simulink model "Trimmodel"  (R2023b)
settings: Solver=ode4  StartTime=0.0  StopTime=100  FixedStep=1e-3  RelTol=1e-3
undefined symbols (not defined in the file or in its folder): Aeroparams, Aircraftparams, Atmosphereparams, Inertiaconstants, Initialconds, Propparams
libraries: simulink_extras x25
(part 2 of 3)

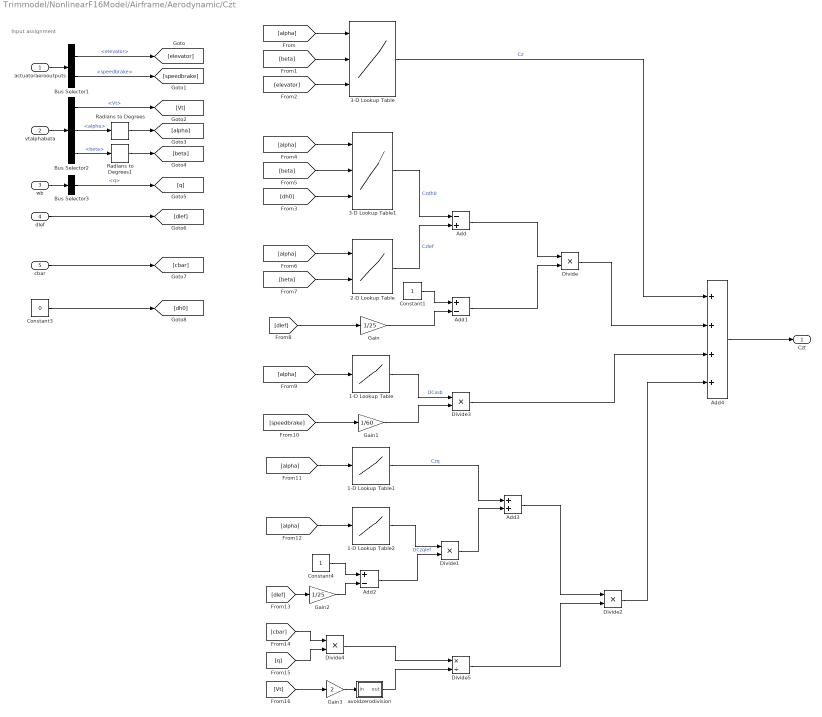
== system Trimmodel/NonlinearF16Model/Airframe/Aerodynamic/Czt ==
  note: Input assignment
  actuatoraerooutputs : Inport
  vtalphabeta : Inport  Port=2
  wb : Inport  Port=3
  dlef : Inport  Port=4
  cbar : Inport  Port=5
  1-D Lookup Table : Lookup_n-D  NumberOfTableDimensions=1  BreakpointsForDimension1=Aeroparams.alpha  Table=Aeroparams.DCzsb  InternalRulePriority=Speed  RndMeth=Simplest
  1-D Lookup Table1 : Lookup_n-D  NumberOfTableDimensions=1  BreakpointsForDimension1=Aeroparams.alpha  Table=Aeroparams.Czq  InternalRulePriority=Speed  RndMeth=Simplest
  1-D Lookup Table2 : Lookup_n-D  NumberOfTableDimensions=1  BreakpointsForDimension1=Aeroparams.alpha(1:14)  Table=Aeroparams.DCzqlef  InternalRulePriority=Speed  RndMeth=Simplest
  2-D Lookup Table : Lookup_n-D  BreakpointsForDimension1=Aeroparams.alpha(1:14)  BreakpointsForDimension2=Aeroparams.beta  Table=Aeroparams.Czlef  InternalRulePriority=Speed  RndMeth=Simplest
      settings: InputPortMap=u0,u1
  3-D Lookup Table : Lookup_n-D  NumberOfTableDimensions=3  BreakpointsForDimension1=Aeroparams.alpha  BreakpointsForDimension2=Aeroparams.beta  BreakpointsForDimension3=Aeroparams.dh  Table=Aeroparams.Cz  InternalRulePriority=Speed  RndMeth=Simplest
      settings: InputPortMap=u0,u1,u2
  3-D Lookup Table1 : Lookup_n-D  NumberOfTableDimensions=3  BreakpointsForDimension1=Aeroparams.alpha  BreakpointsForDimension2=Aeroparams.beta  BreakpointsForDimension3=Aeroparams.dh  Table=Aeroparams.Cz  InternalRulePriority=Speed  RndMeth=Simplest
      settings: InputPortMap=u0,u1,u2
  Add : Sum  Inputs=-+
  Add1 : Sum  Inputs=+-
  Add2 : Sum  Inputs=+-
  Add3 : Sum
  Add4 : Sum  Inputs=++++
  Bus Selector1 : BusSelector  OutputSignals=elevator,speedbrake
  Bus Selector2 : BusSelector  OutputSignals=Vt,alpha,beta
  Bus Selector3 : BusSelector  OutputSignals=q
  Constant1 : Constant
  Constant3 : Constant  Value=0
  Constant4 : Constant
  Divide{,1..4} (5 alike) : Product  Inputs=**
  Divide5 : Product  Inputs=*/
  Gain : Gain  Gain=1/25
  Gain1 : Gain  Gain=1/60
  Gain2 : Gain  Gain=1/25
  Gain3 : Gain  Gain=2
  Radians to Degrees : simulink_extras/Transformations/Radians to Degrees
  Radians to Degrees1 : simulink_extras/Transformations/Radians to Degrees
  avoidzerodivision : Subsystem
  Czt : Outport
  wires:
  Add4/1 -> Czt/1
  Divide2/1 -> Add4/4
  Divide3/1 -> Add4/3
  Divide5/1 -> Divide2/2
  Gain3/1 -> avoidzerodivision/1(in)
  Divide4/1 -> Divide5/1
  [Vt] -> Gain3/1
  [q] -> Divide4/2
  [cbar] -> Divide4/1
  Add3/1 -> Divide2/1
  Divide1/1 -> Add3/2
  1-D Lookup Table1/1 -> Add3/1  "Czq"
  Add2/1 -> Divide1/2
  1-D Lookup Table2/1 -> Divide1/1  "DCzqlef"
  Constant4/1 -> Add2/1
  Gain2/1 -> Add2/2
  [dlef] -> Gain2/1
  [alpha] -> 1-D Lookup Table2/1
  [alpha] -> 1-D Lookup Table1/1
  Gain1/1 -> Divide3/2
  1-D Lookup Table/1 -> Divide3/1  "DCxsb"
  [speedbrake] -> Gain1/1
  [alpha] -> 1-D Lookup Table/1
  [dlef] -> Gain/1
  [beta] -> 2-D Lookup Table/2
  [alpha] -> 2-D Lookup Table/1
  [alpha] -> 3-D Lookup Table1/1
  [beta] -> 3-D Lookup Table1/2
  Constant3/1 -> [dh0]
  [elevator] -> 3-D Lookup Table/3
  [beta] -> 3-D Lookup Table/2
  [alpha] -> 3-D Lookup Table/1
  dlef/1 -> [dlef]
  Bus Selector3/1 -> [q]  "<q>"
  Bus Selector2/3 -> Radians to Degrees1/1  "<beta>"
  Bus Selector2/2 -> Radians to Degrees/1  "<alpha>"
  Bus Selector2/1 -> [Vt]  "<Vt>"
  Bus Selector1/2 -> [speedbrake]  "<speedbrake>"
  Bus Selector1/1 -> [elevator]  "<elevator>"
  Divide/1 -> Add4/2
  Add1/1 -> Divide/2
  Add/1 -> Divide/1
  Gain/1 -> Add1/2
  Constant1/1 -> Add1/1
  3-D Lookup Table1/1 -> Add/1  "Czdh0"
  [dh0] -> 3-D Lookup Table1/3
  2-D Lookup Table/1 -> Add/2  "Czlef"
  3-D Lookup Table/1 -> Add4/1  "Cz"
  wb/1 -> Bus Selector3/1
  vtalphabeta/1 -> Bus Selector2/1
  actuatoraerooutputs/1 -> Bus Selector1/1
  cbar/1 -> [cbar]
  avoidzerodivision/1(out) -> Divide5/2
  Radians to Degrees/1 -> [alpha]
  Radians to Degrees1/1 -> [beta]

== system Trimmodel/NonlinearF16Model/Airframe/Aerodynamic/aeromodelcombineforcesandmoments ==
  Xa : Inport
  Za : Inport  Port=2
  Ma : Inport  Port=3
  Ya : Inport  Port=4
  Na : Inport  Port=5
  La : Inport  Port=6
  Outport : Outport
  Outport1 : Outport  Port=2
  Outport2 : Outport  Port=3
  Outport3 : Outport  Port=4
  Outport4 : Outport  Port=5
  Outport5 : Outport  Port=6
  wires:
  Ya/1 -> Outport1/1  "Ya"
  Xa/1 -> Outport/1  "Xa"
  Za/1 -> Outport2/1  "Za"
  La/1 -> Outport3/1  "La"
  Ma/1 -> Outport4/1  "Ma"
  Na/1 -> Outport5/1  "Na"

== system Trimmodel/NonlinearF16Model/Airframe/Aerodynamic/dlef ==
  vtalphabeta : Inport
  pressure : Inport  Port=2
  Add : Sum  Inputs=+-+
  Bus Selector : BusSelector  OutputSignals=alpha
  Bus Selector1 : BusSelector  OutputSignals=qbar,Ps
  Constant : Constant  Value=1.45
  Divide : Product  Inputs=*/
  Flapactuator : TransferFcn  Denominator=[0.136 1]
  Gain : Gain  Gain=1.38
  Gain1 : Gain  Gain=9.05
  Radians to Degrees : simulink_extras/Transformations/Radians to Degrees
  Rate Limiter : RateLimiter  RisingSlewLimit=25  FallingSlewLimit=-25
  Saturation : Saturate  UpperLimit=25  LowerLimit=0
  Transfer Fcn : TransferFcn  Numerator=[2 7.25]  Denominator=[1 7.25]
  avoidzerodivision : Subsystem
  dlef : Outport
  wires:
  vtalphabeta/1 -> Bus Selector/1
  pressure/1 -> Bus Selector1/1
  Bus Selector1/1 -> Divide/1  "<qbar>"
  Bus Selector1/2 -> avoidzerodivision/1(in)  "<Ps>"
  Bus Selector/1 -> Radians to Degrees/1  "<alpha>"
  Gain/1 -> Transfer Fcn/1
  Divide/1 -> Gain1/1
  Gain1/1 -> Add/2
  Transfer Fcn/1 -> Add/1
  Constant/1 -> Add/3
  Add/1 -> Saturation/1
  Saturation/1 -> Rate Limiter/1
  Rate Limiter/1 -> Flapactuator/1
  avoidzerodivision/1(out) -> Divide/2
  Radians to Degrees/1 -> Gain/1
  Flapactuator/1 -> dlef/1

== system Trimmodel/NonlinearF16Model/Airframe/Aerodynamic/qbarS ==
  pressure : Inport
  S : Inport  Port=2
  Bus Selector1 : BusSelector  OutputSignals=qbar
  Divide : Product  Inputs=**
  qbarS : Outport
  wires:
  pressure/1 -> Bus Selector1/1
  S/1 -> Divide/2  "S"
  Bus Selector1/1 -> Divide/1  "<qbar>"
  Divide/1 -> qbarS/1

== system Trimmodel/NonlinearF16Model/Airframe/Mass/massmodelgb ==
  note: Input assignment
  <phi> : Inport
  <theta> : Inport  Port=2
  <psi> : Inport  Port=3
  Bus Selector2 : BusSelector  OutputSignals=g0
  Constant1 : Constant  Value=Atmosphereparams  OutDataTypeStr=Bus: atmosphereparams
  Constant2 : Constant  Value=0
  Constant3 : Constant  Value=0
  Cos : Trigonometry  Operator=cos
  Cos1 : Trigonometry  Operator=cos
  Cos2 : Trigonometry
  Cos3 : Trigonometry
  Cos4 : Trigonometry  Operator=cos
  Cos5 : Trigonometry
  Firstrow : Subsystem
  Matrix Concatenate : Concatenate  NumInputs=3  Mode=Multidimensional array
  Matrix Multiply : Product  Multiplication=Matrix(*)
  Secondrow : Subsystem
  Thirdrow : Subsystem
  Vector Concatenate : Concatenate  NumInputs=3  Mode=Multidimensional array
  gb : Outport
  wires:
  <theta>/1 -> Cos3/1, Cos/1
  <psi>/1 -> Cos1/1, Cos2/1
  <phi>/1 -> Cos5/1, Cos4/1
  Cos4/1 -> [cosphi]
  Cos5/1 -> [sinphi]
  Cos/1 -> [costheta]
  Cos3/1 -> [sintheta]
  Cos1/1 -> [cospsi]
  Cos2/1 -> [sinpsi]
  Firstrow/1(firstrow) -> Matrix Concatenate/1
  Secondrow/1(secondrow) -> Matrix Concatenate/2
  Thirdrow/1(thirdrow) -> Matrix Concatenate/3
  [sinpsi] -> Secondrow/6(sinpsi)
  [cosphi] -> Thirdrow/1(cosphi)
  [cospsi] -> Secondrow/5(cospsi)
  [sinphi] -> Thirdrow/2(sinphi)
  [cospsi] -> Thirdrow/5(cospsi)
  [sinpsi] -> Firstrow/4(sinpsi)
  [costheta] -> Thirdrow/3(costheta)
  [sinpsi] -> Thirdrow/6(sinpsi)
  [cosphi] -> Secondrow/1(cosphi)
  [sintheta] -> Thirdrow/4(sintheta)
  [sinphi] -> Secondrow/2(sinphi)
  [costheta] -> Firstrow/1(costheta)
  [costheta] -> Secondrow/3(costheta)
  [cospsi] -> Firstrow/3(cospsi)
  [sintheta] -> Secondrow/4(sintheta)
  [sintheta] -> Firstrow/2(sintheta)
  Constant1/1 -> Bus Selector2/1
  Bus Selector2/1 -> [g0]  "<g0>"
  Matrix Concatenate/1 -> Matrix Multiply/1
  Constant3/1 -> Vector Concatenate/2
  Constant2/1 -> Vector Concatenate/1
  [g0] -> Vector Concatenate/3
  Vector Concatenate/1 -> Matrix Multiply/2
  Matrix Multiply/1 -> gb/1  "gxgygz"

== system Trimmodel/NonlinearF16Model/Airframe/Propulsion/Padot ==
  Pc : Inport
  Add : Sum  Inputs=+-
  Bus Selector : BusSelector  OutputSignals=Paic
  Constant : Constant  Value=Initialconds  OutDataTypeStr=Bus: initialconds
  Divide : Product  Inputs=**
  PA : Integrator  InitialConditionSource=external
  propmodeltauPc : Subsystem
  Pa : Outport
  wires:
  PA/1 -> propmodeltauPc/2(Pa), Pa/1, Add/2  "Pa"
  Constant/1 -> Bus Selector/1
  Bus Selector/1 -> PA/2  "<Paic>"
  Pc/1 -> propmodeltauPc/1(Pc)
  propmodeltauPc/2(Outport) -> Add/1
  propmodeltauPc/1(Outport1) -> Divide/1
  Add/1 -> Divide/2
  Divide/1 -> PA/1  "Padot"

== system Trimmodel/NonlinearF16Model/Airframe/Propulsion/Tgear ==
  thrust : Inport
  Add : Sum  Inputs=+-
  Constant : Constant  Value=217.38
  Constant1 : Constant  Value=64.94
  Constant2 : Constant  Value=117.38
  Divide : Product  Inputs=**
  Divide1 : Product  Inputs=**
  Saturation : Saturate  UpperLimit=100  LowerLimit=0
  Switch : Switch  Criteria=u2 > Threshold  Threshold=0.77  SaturateOnIntegerOverflow=off  InputSameDT=off
  Pc : Outport
  wires:
  thrust/1 -> Switch/2, Divide1/1, Divide/2
  Constant/1 -> Divide/1
  Divide1/1 -> Switch/3
  Constant1/1 -> Divide1/2
  Switch/1 -> Saturation/1
  Saturation/1 -> Pc/1
  Divide/1 -> Add/1
  Constant2/1 -> Add/2
  Add/1 -> Switch/1

== system Trimmodel/NonlinearF16Model/Airframe/Propulsion/propmodelTidleTmil ==
  note: Input assignment
  Pa : Inport
  M : Inport  Port=2
  h : Inport  Port=3
  Add : Sum  Inputs=-+
  Add1 : Sum
  Divide : Product  Inputs=**
  Gain : Gain  Gain=1/50
  Tidle : Lookup_n-D  BreakpointsForDimension1=Propparams.M  BreakpointsForDimension2=Propparams.h  Table=Propparams.Tidle  InternalRulePriority=Speed  RndMeth=Simplest
      settings: InputPortMap=u0,u1
  Tmil : Lookup_n-D  BreakpointsForDimension1=Propparams.M  BreakpointsForDimension2=Propparams.h  Table=Propparams.Tmil  InternalRulePriority=Speed  RndMeth=Simplest
      settings: InputPortMap=u0,u1
  Tx : Outport
  wires:
  Tmil/1 -> Add/2
  Tidle/1 -> Add1/1, Add/1
  M/1 -> [M]
  Pa/1 -> [Pa]
  h/1 -> [h]
  [M] -> Tidle/1
  [h] -> Tidle/2
  [M] -> Tmil/1
  [h] -> Tmil/2
  Add/1 -> Divide/1
  [Pa] -> Gain/1
  Gain/1 -> Divide/2
  Divide/1 -> Add1/2
  Add1/1 -> Tx/1

== system Trimmodel/NonlinearF16Model/Airframe/Propulsion/propmodelTmilTmax ==
  note: Input assignment
  M : Inport
  h : Inport  Port=2
  Pa : Inport  Port=3
  Add : Sum  Inputs=-+
  Add1 : Sum
  Add2 : Sum  Inputs=-+
  Constant : Constant  Value=50
  Divide : Product  Inputs=**
  Gain1 : Gain  Gain=1/50
  Tmax : Lookup_n-D  BreakpointsForDimension1=Propparams.M  BreakpointsForDimension2=Propparams.h  Table=Propparams.Tmax  InternalRulePriority=Speed  RndMeth=Simplest
      settings: InputPortMap=u0,u1
  Tmil : Lookup_n-D  BreakpointsForDimension1=Propparams.M  BreakpointsForDimension2=Propparams.h  Table=Propparams.Tmil  InternalRulePriority=Speed  RndMeth=Simplest
      settings: InputPortMap=u0,u1
  Tx : Outport
  wires:
  Add1/1 -> Tx/1
  Divide/1 -> Add1/2
  Gain1/1 -> Divide/2
  [Pa] -> Add2/2
  Add/1 -> Divide/1
  [h] -> Tmax/2
  [M] -> Tmax/1
  [h] -> Tmil/2
  [M] -> Tmil/1
  h/1 -> [h]
  Pa/1 -> [Pa]
  M/1 -> [M]
  Tmil/1 -> Add/1, Add1/1
  Tmax/1 -> Add/2
  Constant/1 -> Add2/1
  Add2/1 -> Gain1/1

== system Trimmodel/NonlinearF16Model/Simframe/Environmentmodel/Vtalphabeta ==
  note: Input assignment
  disturbances : Inport
  bodyvelocities : Inport  Port=2
  Add : Sum  Inputs=-+
  Add1 : Sum  Inputs=-+
  Add2 : Sum  Inputs=-+
  Add3 : Sum  Inputs=+++
  Asin : Trigonometry  Operator=asin
  Atan2 : Trigonometry  Operator=atan2
  Bus Selector : BusSelector  OutputSignals=windz,windy,windx
  Bus Selector1 : BusSelector  OutputSignals=u,v,w
  Divide : Product  Inputs=*/
  Square : Math  Operator=square
  Square Root : Sqrt
  Square1 : Math  Operator=square
  Square2 : Math  Operator=square
  avoidzerodivision : Subsystem
  Vt : Outport
  alpha : Outport  Port=2
  beta : Outport  Port=3
  wires:
  avoidzerodivision/1(out) -> Divide/2
  Asin/1 -> beta/1  "beta"
  Divide/1 -> Asin/1
  [vt] -> Divide/1
  Atan2/1 -> alpha/1  "alpha"
  [ut] -> Atan2/2
  [wt] -> Atan2/1
  Square Root/1 -> avoidzerodivision/1(in), Vt/1  "Vt"
  Add3/1 -> Square Root/1
  Square2/1 -> Add3/3
  Square/1 -> Add3/1
  Square1/1 -> Add3/2
  [wt] -> Square2/1
  [vt] -> Square1/1
  [ut] -> Square/1
  Add2/1 -> [wt]
  Add1/1 -> [vt]
  Add/1 -> [ut]
  Bus Selector/3 -> Add/1  "<windx>"
  Bus Selector/2 -> Add1/1  "<windy>"
  Bus Selector/1 -> Add2/1  "<windz>"
  Bus Selector1/3 -> Add2/2  "<w>"
  Bus Selector1/2 -> Add1/2  "<v>"
  Bus Selector1/1 -> Add/2  "<u>"
  bodyvelocities/1 -> Bus Selector1/1
  disturbances/1 -> Bus Selector/1

== system Trimmodel/NonlinearF16Model/Simframe/Environmentmodel/envmodelTM ==
  note: Input assignment
  T0 : Inport
  L : Inport  Port=2
  h : Inport  Port=3
  gamma : Inport  Port=4
  R : Inport  Port=5
  Vt : Inport  Port=6
  Add : Sum  Inputs=+-
  Add1 : Sum  Inputs=+-
  Constant1 : Constant  Value=11000
  Divide : Product  Inputs=**
  Divide1 : Product  Inputs=**
  Divide15 : Product  Inputs=*/
  Divide2 : Product  Inputs=***
  Square Root : Sqrt
  Switch : Switch  Threshold=11000  SaturateOnIntegerOverflow=off  InputSameDT=off
  T : Outport
  M : Outport  Port=2
  wires:
  gamma/1 -> Divide2/2  "gamma"
  R/1 -> Divide2/3  "R"
  Square Root/1 -> Divide15/2  "a"
  Vt/1 -> Divide15/1
  Divide2/1 -> Square Root/1
  Divide15/1 -> M/1  "M"
  Switch/1 -> Divide2/1, T/1  "T"
  h/1 -> [h]
  L/1 -> [L]
  T0/1 -> [T0]
  [h] -> Switch/2
  Divide/1 -> Add/2
  Divide1/1 -> Add1/2
  Add/1 -> Switch/1  "T11"
  Constant1/1 -> Divide/2
  [T0] -> Add1/1
  [T0] -> Add/1
  [h] -> Divide1/2
  [L] -> Divide/1
  [L] -> Divide1/1
  Add1/1 -> Switch/3  "T"

== system Trimmodel/NonlinearF16Model/Simframe/Environmentmodel/envmodelqbarPs ==
  rho : Inport
  R : Inport  Port=2
  T : Inport  Port=3
  Vt : Inport  Port=4
  Constant3 : Constant  Value=1/2
  Divide13 : Product  Inputs=***
  Divide14 : Product  Inputs=***
  Square : Math  Operator=square
  qbar : Outport
  Ps : Outport  Port=2
  wires:
  Constant3/1 -> Divide14/1
  Square/1 -> Divide14/2
  T/1 -> Divide13/3
  rho/1 -> Divide14/3, Divide13/1
  R/1 -> Divide13/2
  Divide13/1 -> Ps/1  "Ps"
  Vt/1 -> Square/1
  Divide14/1 -> qbar/1  "qbar"

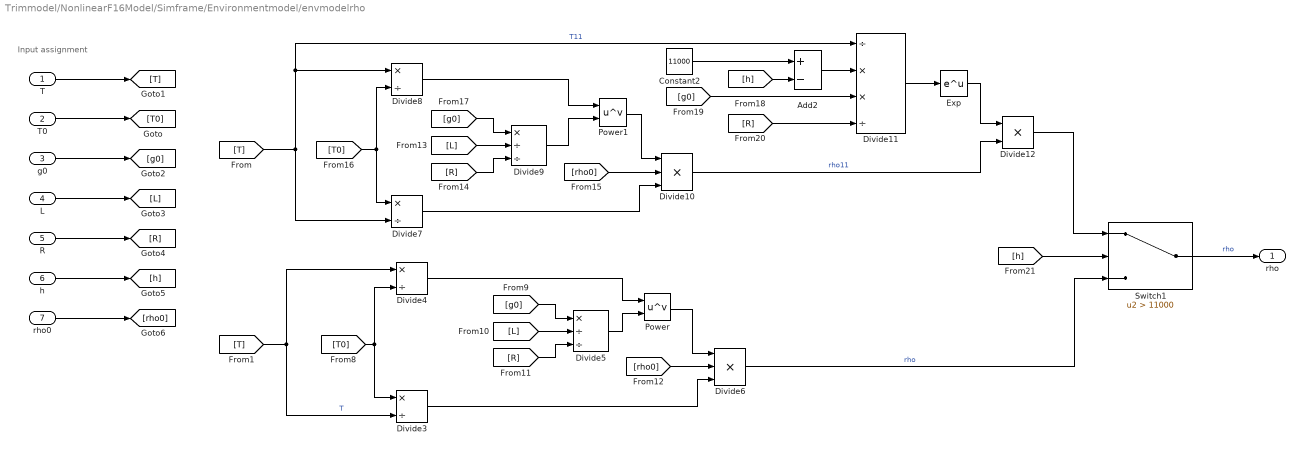
== system Trimmodel/NonlinearF16Model/Simframe/Environmentmodel/envmodelrho ==
  note: Input assignment
  T : Inport
  T0 : Inport  Port=2
  g0 : Inport  Port=3
  L : Inport  Port=4
  R : Inport  Port=5
  h : Inport  Port=6
  rho0 : Inport  Port=7
  Add2 : Sum  Inputs=+-
  Constant2 : Constant  Value=11000
  Divide10 : Product  Inputs=***
  Divide11 : Product  Inputs=/**/
  Divide12 : Product  Inputs=**
  Divide{3..4,7..8} (4 alike) : Product  Inputs=*/
  Divide5 : Product  Inputs=*//
  Divide6 : Product  Inputs=***
  Divide9 : Product  Inputs=*//
  Exp : Math
  Power : Math  Operator=pow
  Power1 : Math  Operator=pow
  Switch1 : Switch  Criteria=u2 > Threshold  Threshold=11000  SaturateOnIntegerOverflow=off  InputSameDT=off
  rho : Outport
  wires:
  Switch1/1 -> rho/1  "rho"
  [h] -> Switch1/2
  rho0/1 -> [rho0]
  h/1 -> [h]
  R/1 -> [R]
  L/1 -> [L]
  g0/1 -> [g0]
  T/1 -> [T]
  T0/1 -> [T0]
  Divide4/1 -> Power/1
  [T0] -> Divide3/1, Divide4/2
  [L] -> Divide5/2
  [g0] -> Divide5/1
  Divide3/1 -> Divide6/3
  [rho0] -> Divide6/2
  [T] -> Divide3/2, Divide4/1  "T"
  Divide6/1 -> Switch1/3  "rho"
  Divide5/1 -> Power/2
  [R] -> Divide5/3
  Power/1 -> Divide6/1
  Exp/1 -> Divide12/1
  Add2/1 -> Divide11/2
  Divide11/1 -> Exp/1
  [g0] -> Divide9/1
  [T] -> Divide7/2, Divide8/1, Divide11/1  "T11"
  [rho0] -> Divide10/2
  [L] -> Divide9/2
  Constant2/1 -> Add2/1
  Divide8/1 -> Power1/1
  Divide9/1 -> Power1/2
  [R] -> Divide11/4
  [R] -> Divide9/3
  Divide10/1 -> Divide12/2  "rho11"
  [T0] -> Divide7/1, Divide8/2
  Power1/1 -> Divide10/1
  [h] -> Add2/2
  [g0] -> Divide11/3
  Divide7/1 -> Divide10/3
  Divide12/1 -> Switch1/1

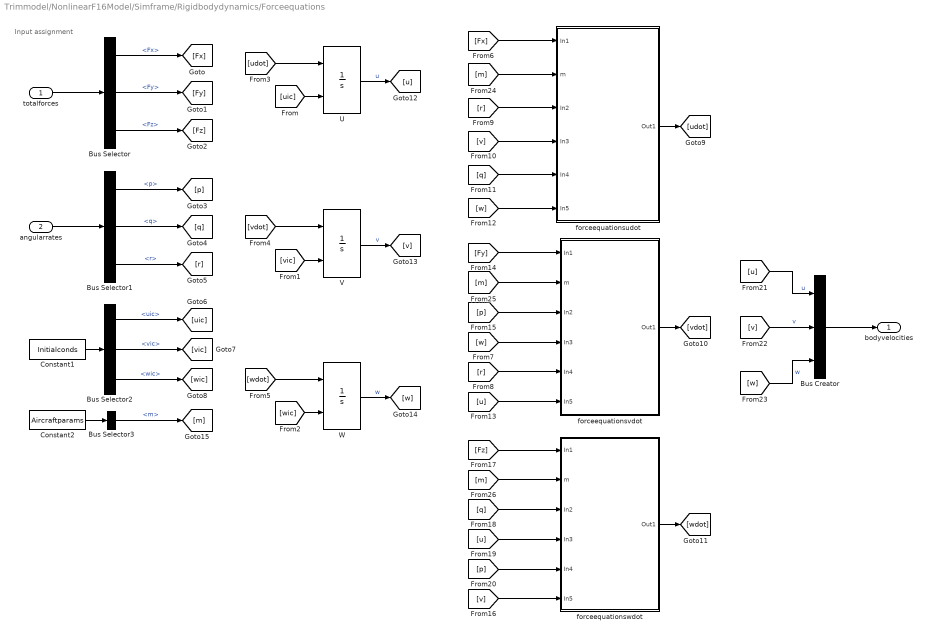
== system Trimmodel/NonlinearF16Model/Simframe/Rigidbodydynamics/Forceequations ==
  note: Input assignment
  totalforces : Inport
  angularrates : Inport  Port=2
  Bus Creator : BusCreator  Inputs=3  OutDataTypeStr=Bus: bodyvelocities
  Bus Selector : BusSelector  OutputSignals=Fx,Fy,Fz
  Bus Selector1 : BusSelector  OutputSignals=p,q,r
  Bus Selector2 : BusSelector  OutputSignals=uic,vic,wic
  Bus Selector3 : BusSelector  OutputSignals=m
  Constant1 : Constant  Value=Initialconds  OutDataTypeStr=Bus: initialconds
  Constant2 : Constant  Value=Aircraftparams  OutDataTypeStr=Bus: aircraftparams
  U : Integrator  InitialConditionSource=external
  V : Integrator  InitialConditionSource=external
  W : Integrator  InitialConditionSource=external
  forceequationsudot : Subsystem
  forceequationsvdot : Subsystem
  forceequationswdot : Subsystem
  bodyvelocities : Outport  OutDataTypeStr=Bus: bodyvelocities
  wires:
  totalforces/1 -> Bus Selector/1
  angularrates/1 -> Bus Selector1/1
  Bus Selector/1 -> [Fx]  "<Fx>"
  Bus Selector/2 -> [Fy]  "<Fy>"
  Bus Selector/3 -> [Fz]  "<Fz>"
  Bus Selector1/1 -> [p]  "<p>"
  Bus Selector1/2 -> [q]  "<q>"
  Bus Selector1/3 -> [r]  "<r>"
  Constant1/1 -> Bus Selector2/1
  Bus Selector2/1 -> [uic]  "<uic>"
  Bus Selector2/2 -> [vic]  "<vic>"
  Bus Selector2/3 -> [wic]  "<wic>"
  [uic] -> U/2
  [vic] -> V/2
  [wic] -> W/2
  forceequationsudot/1(Out1) -> [udot]
  [udot] -> U/1
  [vdot] -> V/1
  [wdot] -> W/1
  U/1 -> [u]  "u"
  V/1 -> [v]  "v"
  W/1 -> [w]  "w"
  [Fx] -> forceequationsudot/1(In1)
  [r] -> forceequationsudot/3(In2)
  [v] -> forceequationsudot/4(In3)
  [q] -> forceequationsudot/5(In4)
  [w] -> forceequationsudot/6(In5)
  [u] -> forceequationsvdot/6(In5)
  [r] -> forceequationsvdot/5(In4)
  [w] -> forceequationsvdot/4(In3)
  [p] -> forceequationsvdot/3(In2)
  [Fy] -> forceequationsvdot/1(In1)
  forceequationsvdot/1(Out1) -> [vdot]
  forceequationswdot/1(Out1) -> [wdot]
  [Fz] -> forceequationswdot/1(In1)
  [q] -> forceequationswdot/3(In2)
  [u] -> forceequationswdot/4(In3)
  [p] -> forceequationswdot/5(In4)
  [v] -> forceequationswdot/6(In5)
  [v] -> Bus Creator/2  "v"
  [u] -> Bus Creator/1  "u"
  [w] -> Bus Creator/3  "w"
  Bus Creator/1 -> bodyvelocities/1
  Constant2/1 -> Bus Selector3/1
  Bus Selector3/1 -> [m]  "<m>"
  [m] -> forceequationsudot/2(m)
  [m] -> forceequationsvdot/2(m)
  [m] -> forceequationswdot/2(m)

== system Trimmodel/NonlinearF16Model/Simframe/Rigidbodydynamics/Kinematicequations ==
  note: Input assignment
  angularrates : Inport
  Bus Creator : BusCreator  Inputs=3  OutDataTypeStr=Bus: eulerangles
  Bus Selector1 : BusSelector  OutputSignals=phiic,thetaic,psiic
  Constant : Constant  Value=Initialconds  OutDataTypeStr=Bus: initialconds
  Eulerlimitations : Subsystem
  PHI : Integrator  InitialConditionSource=external  WrapState=on
  PSI : Integrator  InitialConditionSource=external  WrapState=on
  THETA : Integrator  InitialConditionSource=external  WrapState=on
  kinematicequationseulerdot : Subsystem
  eulerangles : Outport  OutDataTypeStr=Bus: eulerangles
  wires:
  Eulerlimitations/3(Outport1) -> Bus Creator/3
  Eulerlimitations/1(<phi>) -> Bus Creator/1
  Eulerlimitations/2(Outport) -> Bus Creator/2
  [psi] -> Eulerlimitations/3(psi)
  [theta] -> Eulerlimitations/2(theta)
  [phi] -> Eulerlimitations/1(phi)
  PSI/1 -> [psi]  "psi"
  angularrates/1 -> kinematicequationseulerdot/2(angularrates)
  kinematicequationseulerdot/3(psidot) -> PSI/1
  kinematicequationseulerdot/2(thetadot) -> THETA/1
  kinematicequationseulerdot/1(phidot) -> PHI/1
  THETA/1 -> [theta], kinematicequationseulerdot/3(theta)  "theta"
  PHI/1 -> kinematicequationseulerdot/1(phi), [phi]  "phi"
  Bus Creator/1 -> eulerangles/1
  [psiic] -> PSI/2
  [thetaic] -> THETA/2
  [phiic] -> PHI/2
  Bus Selector1/3 -> [psiic]  "<psiic>"
  Bus Selector1/2 -> [thetaic]  "<thetaic>"
  Bus Selector1/1 -> [phiic]  "<phiic>"
  Constant/1 -> Bus Selector1/1

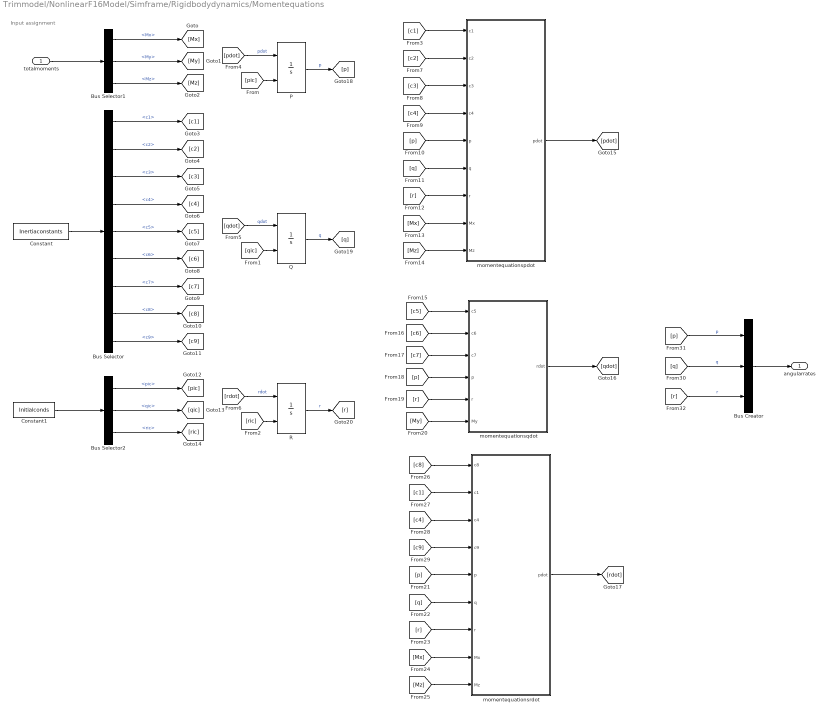
== system Trimmodel/NonlinearF16Model/Simframe/Rigidbodydynamics/Momentequations ==
  note: Input assignment
  totalmoments : Inport
  Bus Creator : BusCreator  Inputs=3  OutDataTypeStr=Bus: angularrates
  Bus Selector : BusSelector  OutputSignals=c1,c2,c3,c4,c5,c6,c7,c8,c9
  Bus Selector1 : BusSelector  OutputSignals=Mx,My,Mz
  Bus Selector2 : BusSelector  OutputSignals=pic,qic,ric
  Constant : Constant  Value=Inertiaconstants  OutDataTypeStr=Bus: inertiaconstants
  Constant1 : Constant  Value=Initialconds  OutDataTypeStr=Bus: initialconds
  P : Integrator  InitialConditionSource=external
  Q : Integrator  InitialConditionSource=external
  R : Integrator  InitialConditionSource=external
  momentequationspdot : Subsystem
  momentequationsqdot : Subsystem
  momentequationsrdot : Subsystem
  angularrates : Outport  OutDataTypeStr=Bus: angularrates
  wires:
  Constant/1 -> Bus Selector/1
  totalmoments/1 -> Bus Selector1/1
  Bus Selector1/1 -> [Mx]  "<Mx>"
  Bus Selector1/2 -> [My]  "<My>"
  Bus Selector1/3 -> [Mz]  "<Mz>"
  Bus Selector/1 -> [c1]  "<c1>"
  Bus Selector/2 -> [c2]  "<c2>"
  Bus Selector/3 -> [c3]  "<c3>"
  Bus Selector/4 -> [c4]  "<c4>"
  Bus Selector/5 -> [c5]  "<c5>"
  Bus Selector/6 -> [c6]  "<c6>"
  Bus Selector/7 -> [c7]  "<c7>"
  Bus Selector/8 -> [c8]  "<c8>"
  Bus Selector/9 -> [c9]  "<c9>"
  Constant1/1 -> Bus Selector2/1
  Bus Selector2/1 -> [pic]  "<pic>"
  Bus Selector2/2 -> [qic]  "<qic>"
  Bus Selector2/3 -> [ric]  "<ric>"
  [pdot] -> P/1  "pdot"
  [qdot] -> Q/1  "qdot"
  [rdot] -> R/1  "rdot"
  [pic] -> P/2
  [qic] -> Q/2
  [ric] -> R/2
  momentequationspdot/1(pdot) -> [pdot]
  momentequationsqdot/1(rdot) -> [qdot]
  P/1 -> [p]  "p"
  Q/1 -> [q]  "q"
  R/1 -> [r]  "r"
  [c1] -> momentequationspdot/1(c1)
  [c2] -> momentequationspdot/2(c2)
  [c3] -> momentequationspdot/3(c3)
  [c4] -> momentequationspdot/4(c4)
  [p] -> momentequationspdot/5(p)
  [q] -> momentequationspdot/6(q)
  [r] -> momentequationspdot/7(r)
  [Mx] -> momentequationspdot/8(Mx)
  [Mz] -> momentequationspdot/9(Mz)
  [c5] -> momentequationsqdot/1(c5)
  [c6] -> momentequationsqdot/2(c6)
  [c7] -> momentequationsqdot/3(c7)
  [p] -> momentequationsqdot/4(p)
  [r] -> momentequationsqdot/5(r)
  [My] -> momentequationsqdot/6(My)
  [Mz] -> momentequationsrdot/9(Mz)
  [Mx] -> momentequationsrdot/8(Mx)
  [r] -> momentequationsrdot/7(r)
  [q] -> momentequationsrdot/6(q)
  [p] -> momentequationsrdot/5(p)
  [c9] -> momentequationsrdot/4(c9)
  [c4] -> momentequationsrdot/3(c4)
  [c1] -> momentequationsrdot/2(c1)
  [c8] -> momentequationsrdot/1(c8)
  momentequationsrdot/1(pdot) -> [rdot]
  [q] -> Bus Creator/2  "q"
  [p] -> Bus Creator/1  "p"
  [r] -> Bus Creator/3  "r"
  Bus Creator/1 -> angularrates/1

== system Trimmodel/NonlinearF16Model/Simframe/Rigidbodydynamics/Navigationequations ==
  note: Input assignment
  bodyvelocities : Inport
  eulerangles : Inport  Port=2
  Bus Creator : BusCreator  Inputs=3  OutDataTypeStr=Bus: positions
  Bus Selector : BusSelector  OutputSignals=u,v,w
  Bus Selector1 : BusSelector  OutputSignals=phi,theta,psi
  Bus Selector2 : BusSelector  OutputSignals=xeic,yeic,zeic
  Constant : Constant  Value=Initialconds  OutDataTypeStr=Bus: initialconds
  Matrix Multiply : Product  Multiplication=Matrix(*)
  Selector : Selector  InputPortWidth=3  IndexOptions=Index vector (dialog)  Indices=1  OutputSizes=1
  Selector1 : Selector  InputPortWidth=3  IndexOptions=Index vector (dialog)  Indices=2  OutputSizes=1
  Selector2 : Selector  InputPortWidth=3  IndexOptions=Index vector (dialog)  Indices=3  OutputSizes=1
  Vector Concatenate : Concatenate  NumInputs=3  Mode=Multidimensional array
  XE : Integrator  InitialConditionSource=external
  YE : Integrator  InitialConditionSource=external
  ZE : Integrator  InitialConditionSource=external
  navigationequationstfmatrix : Subsystem
  positions : Outport  OutDataTypeStr=Bus: positions
  wires:
  bodyvelocities/1 -> Bus Selector/1
  Bus Selector1/2 -> navigationequationstfmatrix/2(<theta>)  "<theta>"
  Bus Selector1/1 -> navigationequationstfmatrix/1(<phi>)  "<phi>"
  Bus Selector1/3 -> navigationequationstfmatrix/3(<psi>)  "<psi>"
  Constant/1 -> Bus Selector2/1
  eulerangles/1 -> Bus Selector1/1
  Bus Selector/2 -> Vector Concatenate/2  "<v>"
  Bus Selector/3 -> Vector Concatenate/3  "<w>"
  Bus Selector/1 -> Vector Concatenate/1  "<u>"
  navigationequationstfmatrix/1(transformationmatrix) -> Matrix Multiply/1
  Vector Concatenate/1 -> Matrix Multiply/2
  Matrix Multiply/1 -> Selector2/1, Selector1/1, Selector/1
  Bus Selector2/1 -> [xeic]  "<xeic>"
  Bus Selector2/2 -> [yeic]  "<yeic>"
  Bus Selector2/3 -> [zeic]  "<zeic>"
  Selector/1 -> XE/1  "xedot"
  [xeic] -> XE/2
  Selector1/1 -> YE/1  "yedot"
  [yeic] -> YE/2
  Selector2/1 -> ZE/1  "zedot"
  [zeic] -> ZE/2
  YE/1 -> Bus Creator/2  "ye"
  XE/1 -> Bus Creator/1  "xe"
  ZE/1 -> Bus Creator/3  "ze"
  Bus Creator/1 -> positions/1

== system Trimmodel/NonlinearF16Model/Airframe/Aerodynamic/Clt/avoidzerodivision ==
  in : Inport
  Constant : Constant  Value=eps
  Switch : Switch  Criteria=u2 ~= 0  SaturateOnIntegerOverflow=off  InputSameDT=off
  out : Outport
  wires:
  in/1 -> Switch/1, Switch/2
  Constant/1 -> Switch/3
  Switch/1 -> out/1

== system Trimmodel/NonlinearF16Model/Airframe/Aerodynamic/Cmt/avoidzerodivision ==
  in : Inport
  Constant : Constant  Value=eps
  Switch : Switch  Criteria=u2 ~= 0  SaturateOnIntegerOverflow=off  InputSameDT=off
  out : Outport
  wires:
  in/1 -> Switch/1, Switch/2
  Constant/1 -> Switch/3
  Switch/1 -> out/1

== system Trimmodel/NonlinearF16Model/Airframe/Aerodynamic/Cnt/avoidzerodivision ==
  in : Inport
  Constant : Constant  Value=eps
  Switch : Switch  Criteria=u2 ~= 0  SaturateOnIntegerOverflow=off  InputSameDT=off
  out : Outport
  wires:
  in/1 -> Switch/1, Switch/2
  Constant/1 -> Switch/3
  Switch/1 -> out/1

== system Trimmodel/NonlinearF16Model/Airframe/Aerodynamic/Cxt/avoidzerodivision ==
  in : Inport
  Constant : Constant  Value=eps
  Switch : Switch  Criteria=u2 ~= 0  SaturateOnIntegerOverflow=off  InputSameDT=off
  out : Outport
  wires:
  in/1 -> Switch/1, Switch/2
  Constant/1 -> Switch/3
  Switch/1 -> out/1

== system Trimmodel/NonlinearF16Model/Airframe/Aerodynamic/Cyt/avoidzerodivision ==
  in : Inport
  Constant : Constant  Value=eps
  Switch : Switch  Criteria=u2 ~= 0  SaturateOnIntegerOverflow=off  InputSameDT=off
  out : Outport
  wires:
  in/1 -> Switch/1, Switch/2
  Constant/1 -> Switch/3
  Switch/1 -> out/1

== system Trimmodel/NonlinearF16Model/Airframe/Aerodynamic/Czt/avoidzerodivision ==
  in : Inport
  Constant : Constant  Value=eps
  Switch : Switch  Criteria=u2 ~= 0  SaturateOnIntegerOverflow=off  InputSameDT=off
  out : Outport
  wires:
  in/1 -> Switch/1, Switch/2
  Constant/1 -> Switch/3
  Switch/1 -> out/1

== system Trimmodel/NonlinearF16Model/Airframe/Aerodynamic/dlef/avoidzerodivision ==
  in : Inport
  Constant : Constant  Value=eps
  Switch : Switch  Criteria=u2 ~= 0  SaturateOnIntegerOverflow=off  InputSameDT=off
  out : Outport
  wires:
  in/1 -> Switch/1, Switch/2
  Constant/1 -> Switch/3
  Switch/1 -> out/1

== system Trimmodel/NonlinearF16Model/Airframe/Mass/massmodelgb/Firstrow ==
  note: Input assignment
  costheta : Inport
  sintheta : Inport  Port=2
  cospsi : Inport  Port=3
  sinpsi : Inport  Port=4
  Divide : Product  Inputs=**
  Divide2 : Product  Inputs=**
  Gain : Gain  Gain=-1
  Vector Concatenate : Concatenate  NumInputs=3  Mode=Multidimensional array  ConcatenateDimension=2
  firstrow : Outport
  wires:
  costheta/1 -> [costheta]
  sintheta/1 -> [sintheta]
  cospsi/1 -> [cospsi]
  sinpsi/1 -> [sinpsi]
  [costheta] -> Divide/1
  [cospsi] -> Divide/2
  [costheta] -> Divide2/1
  [sinpsi] -> Divide2/2
  [sintheta] -> Gain/1
  Divide/1 -> Vector Concatenate/1
  Divide2/1 -> Vector Concatenate/2
  Gain/1 -> Vector Concatenate/3
  Vector Concatenate/1 -> firstrow/1

== system Trimmodel/NonlinearF16Model/Airframe/Mass/massmodelgb/Secondrow ==
  note: Input assignment
  cosphi : Inport
  sinphi : Inport  Port=2
  costheta : Inport  Port=3
  sintheta : Inport  Port=4
  cospsi : Inport  Port=5
  sinpsi : Inport  Port=6
  Add : Sum  Inputs=+-
  Add1 : Sum
  Divide1 : Product  Inputs=***
  Divide2 : Product  Inputs=**
  Divide3 : Product  Inputs=***
  Divide4 : Product  Inputs=**
  Divide5 : Product  Inputs=**
  Vector Concatenate : Concatenate  NumInputs=3  Mode=Multidimensional array  ConcatenateDimension=2
  secondrow : Outport
  wires:
  costheta/1 -> [costheta]
  sintheta/1 -> [sintheta]
  sinphi/1 -> [sinphi]
  cosphi/1 -> [cosphi]
  cospsi/1 -> [cospsi]
  [sinphi] -> Divide1/1
  [sintheta] -> Divide1/2
  [cospsi] -> Divide1/3
  Divide1/1 -> Add/1
  [cosphi] -> Divide2/1
  [sinpsi] -> Divide2/2
  Divide2/1 -> Add/2
  Divide4/1 -> Add1/2
  [cospsi] -> Divide4/2
  [cosphi] -> Divide4/1
  Divide3/1 -> Add1/1
  [sinpsi] -> Divide3/3
  [sintheta] -> Divide3/2
  [sinphi] -> Divide3/1
  [costheta] -> Divide5/2
  sinpsi/1 -> [sinpsi]
  [sinphi] -> Divide5/1
  Add1/1 -> Vector Concatenate/2
  Add/1 -> Vector Concatenate/1
  Divide5/1 -> Vector Concatenate/3
  Vector Concatenate/1 -> secondrow/1

== system Trimmodel/NonlinearF16Model/Airframe/Mass/massmodelgb/Thirdrow ==
  note: Input assignment
  cosphi : Inport
  sinphi : Inport  Port=2
  costheta : Inport  Port=3
  sintheta : Inport  Port=4
  cospsi : Inport  Port=5
  sinpsi : Inport  Port=6
  Add : Sum
  Add1 : Sum  Inputs=+-
  Divide1 : Product  Inputs=***
  Divide2 : Product  Inputs=**
  Divide3 : Product  Inputs=***
  Divide4 : Product  Inputs=**
  Divide5 : Product  Inputs=**
  Vector Concatenate : Concatenate  NumInputs=3  Mode=Multidimensional array  ConcatenateDimension=2
  thirdrow : Outport
  wires:
  Vector Concatenate/1 -> thirdrow/1
  Divide5/1 -> Vector Concatenate/3
  Add/1 -> Vector Concatenate/1
  Add1/1 -> Vector Concatenate/2
  [cosphi] -> Divide5/1
  cospsi/1 -> [cospsi]
  [costheta] -> Divide5/2
  [cosphi] -> Divide3/1
  [sintheta] -> Divide3/2
  [sinpsi] -> Divide3/3
  Divide3/1 -> Add1/1
  [sinphi] -> Divide4/1
  [cospsi] -> Divide4/2
  Divide4/1 -> Add1/2
  Divide2/1 -> Add/2
  [sinpsi] -> Divide2/2
  [sinphi] -> Divide2/1
  Divide1/1 -> Add/1
  [cospsi] -> Divide1/3
  [sintheta] -> Divide1/2
  [cosphi] -> Divide1/1
  sinpsi/1 -> [sinpsi]
  sinphi/1 -> [sinphi]
  cosphi/1 -> [cosphi]
  sintheta/1 -> [sintheta]
  costheta/1 -> [costheta]

== system Trimmodel/NonlinearF16Model/Airframe/Propulsion/Padot/propmodeltauPc ==
  note: Input assignment
  Pc : Inport
  Pa : Inport  Port=2
  If : If  NumInputs=2  IfExpression="u1 >= 50  & u2 >= 50"  ElseIfExpressions=u1 >= 50 & u2 < 50, u1 < 50 & u2 < 50
  If Action Subsystem : Subsystem
  If Action Subsystem1 : Subsystem
  If Action Subsystem2 : Subsystem
  If Action Subsystem3 : Subsystem
  merge : Subsystem
  Outport1 : Outport
  Outport : Outport  Port=2
  wires:
  merge/2(tau) -> Outport1/1  "tau"
  merge/1(Pc) -> Outport/1  "Pc"
  If Action Subsystem3/2(Out2) -> merge/8(In8)
  If Action Subsystem3/1(Out1) -> merge/7(In7)
  If Action Subsystem2/2(Out3) -> merge/6(In6)
  If Action Subsystem2/1(Out2) -> merge/5(In5)
  If Action Subsystem1/2(Out2) -> merge/4(In4)
  If Action Subsystem1/1(Out1) -> merge/3(In3)
  If Action Subsystem/2(Out2) -> merge/2(In2)
  If Action Subsystem/1(Out1) -> merge/1(In1)
  [Pa] -> If Action Subsystem1/1(Pa)
  [Pc] -> If Action Subsystem2/1(Pc)
  If/1 -> If Action Subsystem/Action
  If/2 -> If Action Subsystem1/Action
  [Pc] -> If/1
  [Pa] -> If/2
  [Pa] -> If Action Subsystem2/2(Pa)
  [Pc] -> If Action Subsystem/1(Pc)
  Pc/1 -> [Pc]
  If/3 -> If Action Subsystem2/Action
  Pa/1 -> [Pa]
  If/4 -> If Action Subsystem3/Action

== system Trimmodel/NonlinearF16Model/Simframe/Environmentmodel/Vtalphabeta/avoidzerodivision ==
  in : Inport
  Constant : Constant  Value=eps
  Switch : Switch  Criteria=u2 ~= 0  SaturateOnIntegerOverflow=off  InputSameDT=off
  out : Outport
  wires:
  Switch/1 -> out/1
  Constant/1 -> Switch/3
  in/1 -> Switch/2, Switch/1

== system Trimmodel/NonlinearF16Model/Simframe/Rigidbodydynamics/Forceequations/forceequationsudot ==
  In1 : Inport
  m : Inport  Port=2
  In2 : Inport  Port=3
  In3 : Inport  Port=4
  In4 : Inport  Port=5
  In5 : Inport  Port=6
  Add : Sum  Inputs=++-
  Divide : Product  Inputs=**
  Divide1 : Product  Inputs=**
  Divide2 : Product  Inputs=*/
  Out1 : Outport
  wires:
  In2/1 -> Divide/1
  In3/1 -> Divide/2
  In4/1 -> Divide1/1
  In5/1 -> Divide1/2
  Divide/1 -> Add/2
  Divide1/1 -> Add/3
  Add/1 -> Out1/1  "udot"
  m/1 -> Divide2/2
  In1/1 -> Divide2/1
  Divide2/1 -> Add/1

== system Trimmodel/NonlinearF16Model/Simframe/Rigidbodydynamics/Forceequations/forceequationsvdot ==
  In1 : Inport
  m : Inport  Port=2
  In2 : Inport  Port=3
  In3 : Inport  Port=4
  In4 : Inport  Port=5
  In5 : Inport  Port=6
  Add : Sum  Inputs=++-
  Divide : Product  Inputs=**
  Divide1 : Product  Inputs=**
  Divide2 : Product  Inputs=*/
  Out1 : Outport
  wires:
  Add/1 -> Out1/1  "vdot"
  Divide1/1 -> Add/3
  Divide/1 -> Add/2
  In5/1 -> Divide1/2
  In4/1 -> Divide1/1
  In3/1 -> Divide/2
  In2/1 -> Divide/1
  m/1 -> Divide2/2
  In1/1 -> Divide2/1
  Divide2/1 -> Add/1

== system Trimmodel/NonlinearF16Model/Simframe/Rigidbodydynamics/Forceequations/forceequationswdot ==
  In1 : Inport
  m : Inport  Port=2
  In2 : Inport  Port=3
  In3 : Inport  Port=4
  In4 : Inport  Port=5
  In5 : Inport  Port=6
  Add : Sum  Inputs=++-
  Divide : Product  Inputs=**
  Divide1 : Product  Inputs=**
  Divide2 : Product  Inputs=*/
  Out1 : Outport
  wires:
  In2/1 -> Divide/1
  In3/1 -> Divide/2
  In4/1 -> Divide1/1
  In5/1 -> Divide1/2
  Divide/1 -> Add/2
  In1/1 -> Divide2/1
  Divide1/1 -> Add/3
  Add/1 -> Out1/1  "wdot"
  m/1 -> Divide2/2
  Divide2/1 -> Add/1

== system Trimmodel/NonlinearF16Model/Simframe/Rigidbodydynamics/Kinematicequations/Eulerlimitations ==
  note: $-\pi <= \phi < \pi \\ -\pi/2 <= \theta <= \pi/2 \\ -\pi <= \psi < \pi \\$
  note: Input assignment
  phi : Inport
  theta : Inport  Port=2
  psi : Inport  Port=3
  Constant1 : Constant  Value=(3/2)*pi
  Constant2 : Constant  Value=(1/2)*pi
  Constant3 : Constant  Value=(-3/2)*pi
  Constant4 : Constant  Value=(-1/2)*pi
  If : If  NumInputs=5  IfExpression=u1 >= u2  ElseIfExpressions=u1 > u3, u1 <= u4, u1 < u5
  If Action Subsystem : Subsystem
  If Action Subsystem1 : Subsystem
  If Action Subsystem2 : Subsystem
  If Action Subsystem3 : Subsystem
  If Action Subsystem4 : Subsystem
  Phi : Subsystem
  Psi : Subsystem
  merge : Subsystem
  <phi> : Outport
  Outport : Outport  Port=2
  Outport1 : Outport  Port=3
  wires:
  [theta] -> If Action Subsystem3/2(theta)
  merge/3(Out3) -> Psi/1(psi)
  [psi] -> If Action Subsystem3/3(psi)
  [theta] -> If Action Subsystem1/2(theta)
  [phi] -> If Action Subsystem1/1(phi)
  [theta] -> If Action Subsystem/2(theta)
  [psi] -> If Action Subsystem1/3(psi)
  merge/1(Out1) -> Phi/1(phi)
  [theta] -> If Action Subsystem2/2(theta)
  [phi] -> If Action Subsystem4/1(phi)
  [psi] -> If Action Subsystem4/3(psi)
  psi/1 -> [psi]
  phi/1 -> [phi]
  [phi] -> If Action Subsystem3/1(phi)
  [theta] -> If Action Subsystem4/2(theta)
  Phi/1(Out1) -> <phi>/1  "phi"
  merge/2(Outport) -> Outport/1  "theta"
  Psi/1(Outport1) -> Outport1/1  "psi"
  [phi] -> If Action Subsystem/1(phi)
  [psi] -> If Action Subsystem/3(psi)
  [phi] -> If Action Subsystem2/1(phi)
  [psi] -> If Action Subsystem2/3(psi)
  If Action Subsystem/1(Out2) -> merge/1(In1)
  If Action Subsystem/2(Out1) -> merge/2(In2)
  If Action Subsystem/3(Out3) -> merge/3(In3)
  If Action Subsystem1/1(Out1) -> merge/4(In4)
  If Action Subsystem1/2(Out2) -> merge/5(In5)
  If Action Subsystem1/3(Out3) -> merge/6(In6)
  If Action Subsystem2/1(Out2) -> merge/7(In7)
  If Action Subsystem2/2(Out1) -> merge/8(In8)
  If Action Subsystem2/3(Out3) -> merge/9(In9)
  If Action Subsystem3/1(Out1) -> merge/10(In10)
  If Action Subsystem3/2(Out2) -> merge/11(In11)
  If Action Subsystem3/3(Out3) -> merge/12(In12)
  If Action Subsystem4/1(Out1) -> merge/13(In13)
  If Action Subsystem4/2(Out2) -> merge/14(In14)
  If Action Subsystem4/3(Out3) -> merge/15(In15)
  theta/1 -> [theta]
  [theta] -> If/1
  Constant1/1 -> If/2
  Constant2/1 -> If/3
  Constant3/1 -> If/4
  Constant4/1 -> If/5
  If/1 -> If Action Subsystem/Action
  If/2 -> If Action Subsystem1/Action
  If/3 -> If Action Subsystem2/Action
  If/4 -> If Action Subsystem3/Action
  If/5 -> If Action Subsystem4/Action

== system Trimmodel/NonlinearF16Model/Simframe/Rigidbodydynamics/Kinematicequations/kinematicequationseulerdot ==
  phi : Inport
  angularrates : Inport  Port=2
  theta : Inport  Port=3
  Avoidsingularity : Subsystem
  Constant : Constant  Value=0
  Cos : Trigonometry  Operator=cos
  Cos1 : Trigonometry
  Gain : Gain  Gain=-1
  Matrix Multiply : Product  Multiplication=Matrix(*)
  Matrix Multiply1 : Product  Multiplication=Matrix(*)
  Selector : Selector  InputPortWidth=3  IndexOptions=Index vector (dialog)  Indices=1  OutputSizes=1
  Selector1 : Selector  InputPortWidth=3  IndexOptions=Index vector (dialog)  Indices=2  OutputSizes=1
  Selector2 : Selector  InputPortWidth=3  IndexOptions=Index vector (dialog)  Indices=3  OutputSizes=1
  Vector Concatenate : Concatenate  NumInputs=3  Mode=Multidimensional array  ConcatenateDimension=2
  kinematicequationstfmatrix : Subsystem
  phidot : Outport
  thetadot : Outport  Port=2
  psidot : Outport  Port=3
  wires:
  Matrix Multiply1/1 -> Avoidsingularity/2(thetadot)
  theta/1 -> Avoidsingularity/1(theta)
  Vector Concatenate/1 -> Matrix Multiply1/1  "secondrowofrotationmatrix"
  Gain/1 -> Vector Concatenate/3
  Cos/1 -> Vector Concatenate/2
  Cos1/1 -> Gain/1
  Constant/1 -> Vector Concatenate/1
  Selector/1 -> phidot/1  "phidot"
  Avoidsingularity/1(Outport) -> kinematicequationstfmatrix/2(<theta>)
  Selector1/1 -> thetadot/1  "thetadot"
  angularrates/1 -> Matrix Multiply1/2, Matrix Multiply/2  "angularrates"
  Selector2/1 -> psidot/1  "psidot"
  Matrix Multiply/1 -> Selector2/1, Selector1/1, Selector/1
  kinematicequationstfmatrix/1(transformationmatrix) -> Matrix Multiply/1
  phi/1 -> Cos/1, Cos1/1, kinematicequationstfmatrix/1(<phi>)

== system Trimmodel/NonlinearF16Model/Simframe/Rigidbodydynamics/Momentequations/momentequationspdot ==
  c1 : Inport
  c2 : Inport  Port=2
  c3 : Inport  Port=3
  c4 : Inport  Port=4
  p : Inport  Port=5
  q : Inport  Port=6
  r : Inport  Port=7
  Mx : Inport  Port=8
  Mz : Inport  Port=9
  Add : Sum
  Add1 : Sum  Inputs=+--
  Divide{,1..4} (5 alike) : Product  Inputs=**
  pdot : Outport
  wires:
  c1/1 -> Divide/1
  p/1 -> Divide/2
  c2/1 -> Divide1/1
  r/1 -> Divide1/2
  Divide/1 -> Add/1
  Divide1/1 -> Add/2
  Add/1 -> Divide2/1
  q/1 -> Divide2/2
  c3/1 -> Divide3/1
  Mx/1 -> Divide3/2
  c4/1 -> Divide4/1
  Mz/1 -> Divide4/2
  Divide3/1 -> Add1/2
  Divide2/1 -> Add1/1
  Divide4/1 -> Add1/3
  Add1/1 -> pdot/1  "pdot"

== system Trimmodel/NonlinearF16Model/Simframe/Rigidbodydynamics/Momentequations/momentequationsqdot ==
  c5 : Inport
  c6 : Inport  Port=2
  c7 : Inport  Port=3
  p : Inport  Port=4
  r : Inport  Port=5
  My : Inport  Port=6
  Add : Sum  Inputs=-+
  Add1 : Sum  Inputs=-++
  Divide : Product  Inputs=**
  Divide1 : Product  Inputs=***
  Divide2 : Product  Inputs=**
  Square : Math  Operator=square
  Square1 : Math  Operator=square
  rdot : Outport
  wires:
  r/1 -> Divide1/2, Square/1
  p/1 -> Divide1/1, Square1/1
  Square/1 -> Add/2
  Square1/1 -> Add/1
  c5/1 -> Divide/1
  Add/1 -> Divide/2
  c6/1 -> Divide1/3
  My/1 -> Divide2/1
  c7/1 -> Divide2/2
  Divide1/1 -> Add1/1
  Divide/1 -> Add1/2
  Divide2/1 -> Add1/3
  Add1/1 -> rdot/1  "qdot"

== system Trimmodel/NonlinearF16Model/Simframe/Rigidbodydynamics/Momentequations/momentequationsrdot ==
  c8 : Inport
  c1 : Inport  Port=2
  c4 : Inport  Port=3
  c9 : Inport  Port=4
  p : Inport  Port=5
  q : Inport  Port=6
  r : Inport  Port=7
  Mx : Inport  Port=8
  Mz : Inport  Port=9
  Add : Sum  Inputs=+-
  Add1 : Sum  Inputs=+--
  Divide{,1..4} (5 alike) : Product  Inputs=**
  pdot : Outport
  wires:
  Add1/1 -> pdot/1  "rdot"
  Divide4/1 -> Add1/3
  Divide2/1 -> Add1/1
  Divide3/1 -> Add1/2
  Mz/1 -> Divide4/2
  c9/1 -> Divide4/1
  Mx/1 -> Divide3/2
  c4/1 -> Divide3/1
  q/1 -> Divide2/2
  Add/1 -> Divide2/1
  Divide1/1 -> Add/2
  Divide/1 -> Add/1
  r/1 -> Divide1/2
  c1/1 -> Divide1/1
  p/1 -> Divide/2
  c8/1 -> Divide/1

== system Trimmodel/NonlinearF16Model/Simframe/Rigidbodydynamics/Navigationequations/navigationequationstfmatrix ==
  note: Input assignment
  <phi> : Inport
  <theta> : Inport  Port=2
  <psi> : Inport  Port=3
  Cos : Trigonometry  Operator=cos
  Cos1 : Trigonometry  Operator=cos
  Cos2 : Trigonometry
  Cos3 : Trigonometry
  Cos4 : Trigonometry  Operator=cos
  Cos5 : Trigonometry
  Matrix Concatenate : Concatenate  NumInputs=3  Mode=Multidimensional array
  firstrow : Subsystem
  secondrow : Subsystem
  thirdrow : Subsystem
  transformationmatrix : Outport
  wires:
  <theta>/1 -> Cos3/1, Cos/1
  <psi>/1 -> Cos1/1, Cos2/1
  <phi>/1 -> Cos5/1, Cos4/1
  Cos4/1 -> [cosphi]
  Cos5/1 -> [sinphi]
  Cos/1 -> [costheta]
  Cos3/1 -> [sintheta]
  Cos1/1 -> [cospsi]
  Cos2/1 -> [sinpsi]
  firstrow/1(firstrow) -> Matrix Concatenate/1
  thirdrow/1(thirdrow) -> Matrix Concatenate/3
  Matrix Concatenate/1 -> transformationmatrix/1
  [sintheta] -> firstrow/4(sintheta)
  [costheta] -> firstrow/3(costheta)
  [sinphi] -> firstrow/2(sinphi)
  [cosphi] -> firstrow/1(cosphi)
  [cospsi] -> firstrow/5(cospsi)
  [sinpsi] -> firstrow/6(sinpsi)
  [sinpsi] -> secondrow/6(sinpsi)
  [cospsi] -> secondrow/5(cospsi)
  [cosphi] -> secondrow/1(cosphi)
  [sinphi] -> secondrow/2(sinphi)
  [costheta] -> secondrow/3(costheta)
  [sintheta] -> secondrow/4(sintheta)
  secondrow/1(secondrow) -> Matrix Concatenate/2
  [cosphi] -> thirdrow/1(cosphi)
  [sinphi] -> thirdrow/2(sinphi)
  [costheta] -> thirdrow/3(costheta)
  [sintheta] -> thirdrow/4(sintheta)

== system Trimmodel/NonlinearF16Model/Airframe/Propulsion/Padot/propmodeltauPc/If Action Subsystem ==
  Pc : Inport
  Action Port : ActionPort  ActionPortLabel="if(u1 >= 50  & u2 >= 50)"
  Constant : Constant  Value=5
  Out1 : Outport
  Out2 : Outport  Port=2
  wires:
  Constant/1 -> Out2/1  "tau"
  Pc/1 -> Out1/1  "Pc"

== system Trimmodel/NonlinearF16Model/Airframe/Propulsion/Padot/propmodeltauPc/If Action Subsystem1 ==
  Pa : Inport
  Action Port : ActionPort  ActionPortLabel=elseif(u1 >= 50 & u2 < 50)
  Add : Sum  Inputs=+-
  Constant : Constant  Value=60
  If : If  IfExpression=u1 <= 25  ElseIfExpressions=u1 >= 50
  If Action Subsystem : Subsystem
  If Action Subsystem1 : Subsystem
  If Action Subsystem2 : Subsystem
  Merge : Merge  Inputs=3
  Out1 : Outport
  Out2 : Outport  Port=2
  wires:
  Merge/1 -> Out2/1  "tau"
  If Action Subsystem2/1(tau) -> Merge/3
  If Action Subsystem1/1(tau) -> Merge/2
  If Action Subsystem/1(tau) -> Merge/1
  If/3 -> If Action Subsystem2/Action
  If/2 -> If Action Subsystem1/Action
  If/1 -> If Action Subsystem/Action
  Add/1 -> If/1, If Action Subsystem2/1(dP)  "dP"
  Pa/1 -> Add/2
  Constant/1 -> Out1/1, Add/1  "Pc"

== system Trimmodel/NonlinearF16Model/Airframe/Propulsion/Padot/propmodeltauPc/If Action Subsystem2 ==
  Pc : Inport
  Pa : Inport  Port=2
  Action Port : ActionPort  ActionPortLabel=elseif( u1 < 50 & u2 < 50)
  Add : Sum  Inputs=+-
  If : If  IfExpression=u1 <= 25  ElseIfExpressions=u1 >= 50
  If Action Subsystem : Subsystem
  If Action Subsystem1 : Subsystem
  If Action Subsystem2 : Subsystem
  Merge : Merge  Inputs=3
  Out2 : Outport
  Out3 : Outport  Port=2
  wires:
  If/1 -> If Action Subsystem/Action
  If Action Subsystem2/1(tau) -> Merge/3
  Add/1 -> If/1, If Action Subsystem2/1(dP)  "dP"
  Merge/1 -> Out3/1  "tau"
  If/3 -> If Action Subsystem2/Action
  If Action Subsystem1/1(tau) -> Merge/2
  If Action Subsystem/1(tau) -> Merge/1
  Pa/1 -> Add/2
  Pc/1 -> Out2/1, Add/1  "Pc"
  If/2 -> If Action Subsystem1/Action

== system Trimmodel/NonlinearF16Model/Airframe/Propulsion/Padot/propmodeltauPc/If Action Subsystem3 ==
  Action Port : ActionPort  ActionPortLabel=else
  Constant : Constant  Value=40
  Constant1 : Constant  Value=5
  Out1 : Outport
  Out2 : Outport  Port=2
  wires:
  Constant1/1 -> Out2/1  "tau"
  Constant/1 -> Out1/1  "Pc"

== system Trimmodel/NonlinearF16Model/Airframe/Propulsion/Padot/propmodeltauPc/merge ==
  In1 : Inport
  In2 : Inport  Port=2
  In3 : Inport  Port=3
  In4 : Inport  Port=4
  In5 : Inport  Port=5
  In6 : Inport  Port=6
  In7 : Inport  Port=7
  In8 : Inport  Port=8
  Merge : Merge  Inputs=4
  Merge1 : Merge  Inputs=4
  Pc : Outport
  tau : Outport  Port=2
  wires:
  Merge1/1 -> tau/1
  Merge/1 -> Pc/1
  In8/1 -> Merge1/4
  In6/1 -> Merge1/3
  In4/1 -> Merge1/2
  In2/1 -> Merge1/1
  In7/1 -> Merge/4
  In5/1 -> Merge/3
  In3/1 -> Merge/2
  In1/1 -> Merge/1

== system Trimmodel/NonlinearF16Model/Simframe/Rigidbodydynamics/Kinematicequations/Eulerlimitations/If Action Subsystem ==
  phi : Inport
  theta : Inport  Port=2
  psi : Inport  Port=3
  Action Port : ActionPort  ActionPortLabel=if(u1 >= u2)
  Add : Sum  Inputs=+-
  Constant : Constant  Value=2*pi
  Out2 : Outport
  Out1 : Outport  Port=2
  Out3 : Outport  Port=3
  wires:
  theta/1 -> Add/1
  Constant/1 -> Add/2
  Add/1 -> Out1/1  "theta"
  phi/1 -> Out2/1  "phi"
  psi/1 -> Out3/1  "psi"

== system Trimmodel/NonlinearF16Model/Simframe/Rigidbodydynamics/Kinematicequations/Eulerlimitations/If Action Subsystem1 ==
  phi : Inport
  theta : Inport  Port=2
  psi : Inport  Port=3
  Action Port : ActionPort  ActionPortLabel=elseif(u1 > u3)
  Add : Sum  Inputs=+-
  Add1 : Sum  Inputs=-+
  Add2 : Sum  Inputs=+-
  Constant : Constant  Value=pi
  Constant1 : Constant  Value=pi
  Constant2 : Constant  Value=pi
  Out1 : Outport
  Out2 : Outport  Port=2
  Out3 : Outport  Port=3
  wires:
  phi/1 -> Add/1
  Constant/1 -> Add/2
  Add/1 -> Out1/1  "phi"
  theta/1 -> Add1/1
  Constant1/1 -> Add1/2
  Add1/1 -> Out2/1  "theta"
  psi/1 -> Add2/1
  Constant2/1 -> Add2/2
  Add2/1 -> Out3/1  "psi"

== system Trimmodel/NonlinearF16Model/Simframe/Rigidbodydynamics/Kinematicequations/Eulerlimitations/If Action Subsystem2 ==
  phi : Inport
  theta : Inport  Port=2
  psi : Inport  Port=3
  Action Port : ActionPort  ActionPortLabel=elseif( u1 <= u4)
  Add : Sum
  Constant : Constant  Value=2*pi
  Out2 : Outport
  Out1 : Outport  Port=2
  Out3 : Outport  Port=3
  wires:
  phi/1 -> Out2/1  "phi"
  theta/1 -> Add/1
  Constant/1 -> Add/2
  psi/1 -> Out3/1  "psi"
  Add/1 -> Out1/1  "theta"

== system Trimmodel/NonlinearF16Model/Simframe/Rigidbodydynamics/Kinematicequations/Eulerlimitations/If Action Subsystem3 ==
  phi : Inport
  theta : Inport  Port=2
  psi : Inport  Port=3
  Action Port : ActionPort  ActionPortLabel=elseif( u1 < u5)
  Add : Sum  Inputs=+-
  Add1 : Sum  Inputs=--
  Add2 : Sum  Inputs=+-
  Constant : Constant  Value=pi
  Constant1 : Constant  Value=pi
  Constant2 : Constant  Value=pi
  Out1 : Outport
  Out2 : Outport  Port=2
  Out3 : Outport  Port=3
  wires:
  Add2/1 -> Out3/1  "psi"
  psi/1 -> Add2/1
  phi/1 -> Add/1
  Constant2/1 -> Add2/2
  Constant1/1 -> Add1/2
  theta/1 -> Add1/1
  Add1/1 -> Out2/1  "theta"
  Constant/1 -> Add/2
  Add/1 -> Out1/1  "phi"

== system Trimmodel/NonlinearF16Model/Simframe/Rigidbodydynamics/Kinematicequations/Eulerlimitations/If Action Subsystem4 ==
  phi : Inport
  theta : Inport  Port=2
  psi : Inport  Port=3
  Action Port : ActionPort  ActionPortLabel=else
  Out1 : Outport
  Out2 : Outport  Port=2
  Out3 : Outport  Port=3
  wires:
  phi/1 -> Out1/1  "phi"
  theta/1 -> Out2/1  "theta"
  psi/1 -> Out3/1  "psi"

== system Trimmodel/NonlinearF16Model/Simframe/Rigidbodydynamics/Kinematicequations/Eulerlimitations/Phi ==
  note: Input assignment
  phi : Inport
  Constant1 : Constant  Value=pi
  Constant2 : Constant  Value=-pi
  If : If  NumInputs=3  IfExpression=u1 >= u2  ElseIfExpressions=u1 < u3
  If Action Subsystem : Subsystem
  If Action Subsystem1 : Subsystem
  If Action Subsystem2 : Subsystem
  Merge : Merge  Inputs=3
  Out1 : Outport
  wires:
  [phi] -> If Action Subsystem1/1(phi)
  [phi] -> If Action Subsystem/1(phi)
  If Action Subsystem/1(Out1) -> Merge/1
  If Action Subsystem1/1(Out1) -> Merge/2
  Merge/1 -> Out1/1  "phi"
  [phi] -> If Action Subsystem2/1(phi)
  If Action Subsystem2/1(Out1) -> Merge/3
  phi/1 -> [phi]
  [phi] -> If/1
  Constant1/1 -> If/2
  Constant2/1 -> If/3
  If/1 -> If Action Subsystem/Action
  If/2 -> If Action Subsystem1/Action
  If/3 -> If Action Subsystem2/Action

== system Trimmodel/NonlinearF16Model/Simframe/Rigidbodydynamics/Kinematicequations/Eulerlimitations/Psi ==
  note: Input assignment
  psi : Inport
  Constant1 : Constant  Value=pi
  Constant2 : Constant  Value=-pi
  If : If  NumInputs=3  IfExpression=u1 >= u2  ElseIfExpressions=u1 < u3
  If Action Subsystem : Subsystem
  If Action Subsystem1 : Subsystem
  If Action Subsystem2 : Subsystem
  Merge : Merge  Inputs=3
  Outport1 : Outport
  wires:
  Merge/1 -> Outport1/1  "psi"
  If Action Subsystem1/1(Out1) -> Merge/2
  If Action Subsystem/1(Out1) -> Merge/1
  [psi] -> If Action Subsystem/1(psi)
  [psi] -> If Action Subsystem1/1(psi)
  [psi] -> If Action Subsystem2/1(psi)
  If Action Subsystem2/1(Out1) -> Merge/3
  psi/1 -> [psi]
  [psi] -> If/1
  Constant1/1 -> If/2
  Constant2/1 -> If/3
  If/1 -> If Action Subsystem/Action
  If/2 -> If Action Subsystem1/Action
  If/3 -> If Action Subsystem2/Action
